simulink model "PWMinverter"  (Simulink 7.3)
settings: Solver=ode23tb  StartTime=0.0  StopTime=0.1  MaxStep=1e-5  RelTol=1e-3
libraries: powerlib x11, simulink x2
settings Model: Creator=viswam  LastModifiedBy=viswam
settings SolverCC: InitialStep=1e-6
settings OptimizationCC: InitFltsAndDblsToZero=on
settings DebuggingCC: SaveWithParameterizedLinksMsg=none  SignalResolutionControl=TryResolveAllWithWarning  MultiTaskDSMMsg=warning  MultiTaskCondExecSysMsg=none
settings RTWCC: IncludeERTFirstTime=on
settings GRTTargetCC: TargetFcnLib=ansi_tfl_tmw.mat

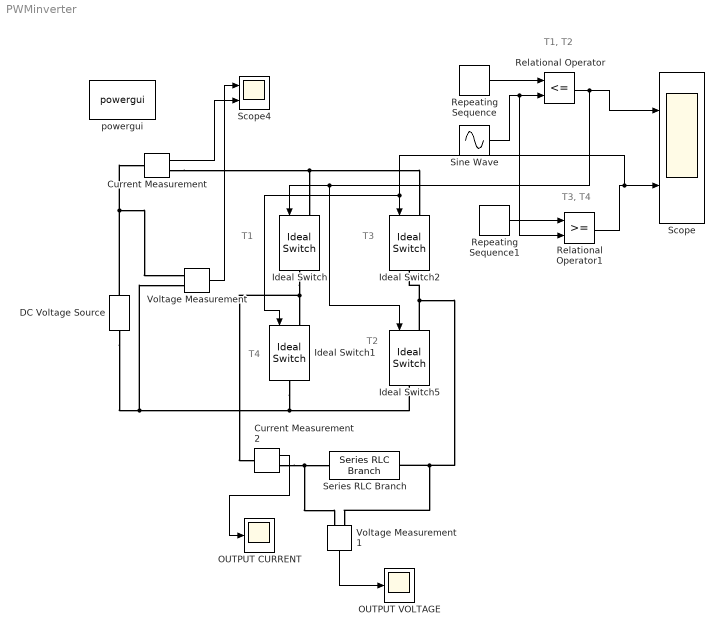
== system PWMinverter ==
  note: T1
  note: T2
  note: T3
  note: T4
  note: T1, T2
  note: T3, T4
  Current Measurement : powerlib/Measurements/Current Measurement  DialogController=POWERSYS.PowerSysDialog  SystemSampleTime=-1  PhasorSimulation=off  OutputType=Complex  PSBequivalent=0
  Current Measurement2 : powerlib/Measurements/Current Measurement  DialogController=POWERSYS.PowerSysDialog  SystemSampleTime=-1  PhasorSimulation=off  OutputType=Complex  PSBequivalent=0
  DC Voltage Source : powerlib/Electrical Sources/DC Voltage Source  DialogController=POWERSYS.PowerSysDialog  SystemSampleTime=-1  Amplitude=300  Measurements=None
  Ideal Switch{,1..2,5} (4 alike) : powerlib/Power Electronics/Ideal Switch  DialogController=POWERSYS.PowerSysDialog  SystemSampleTime=-1  Ron=0.001  Lon=0  IC=0  Rs=1e5  Cs=inf  Measurements=off
  OUTPUT CURRENT : Scope
      settings: TimeRange=0.04  YMin=-50  YMax=50  SaveName=outputcurrent
  OUTPUT VOLTAGE : Scope
      settings: TimeRange=0.04  YMin=-500  YMax=500  SaveName=outputvoltage
  Relational Operator : RelationalOperator  Operator=<=  LogicOutDataTypeMode=boolean  OutDataTypeStr=boolean
  Relational Operator1 : RelationalOperator  LogicOutDataTypeMode=boolean  OutDataTypeStr=boolean
  Repeating Sequence : simulink/Sources/Repeating Sequence  SystemSampleTime=-1  rep_seq_t=[0 0.5e-3 1e-3]  rep_seq_y=[0 1 0]
  Repeating Sequence1 : simulink/Sources/Repeating Sequence  SystemSampleTime=-1  rep_seq_t=[0 0.5e-3 1e-3]  rep_seq_y=[-1 0 -1]
  Scope : Scope  NumInputPorts=2
      settings: TimeRange=0.04  YMin=-5~-5  YMax=5~5
  Scope4 : Scope  NumInputPorts=2
      settings: TimeRange=0.04  YMin=-5~-5  YMax=5~5  SaveName=ScopeData4
  Series RLC Branch : powerlib/Elements/Series RLC Branch  DialogController=POWERSYS.PowerSysDialog  PhysicalDomain=powersysdomain  SubClassName=unknown  LeftPortType=p1  RightPortType=p1  LConnTagsString=__new0  RConnTagsString=__new0  BranchType=R  Resistance=10  Inductance=1e-3  SetiL0=off  InitialCurrent=0  Capacitance=1e-6  Setx0=off  InitialVoltage=0  Measurements=None
  Sine Wave : Sin  Amplitude=1  Bias=0  Frequency=2*pi*50  Phase=0  Samples=10  SampleTime=0  Offset=0
  Voltage Measurement : powerlib/Measurements/Voltage Measurement  DialogController=POWERSYS.PowerSysDialog  SystemSampleTime=-1  PhasorSimulation=off  OutputType=Complex  PSBequivalent=0
  Voltage Measurement1 : powerlib/Measurements/Voltage Measurement  DialogController=POWERSYS.PowerSysDialog  SystemSampleTime=-1  PhasorSimulation=off  OutputType=Complex  PSBequivalent=0
  powergui : powerlib/powergui  Priority=1  SystemSampleTime=-1  SimulationMode=Continuous  SampleTime=50e-6  frequency=60  SPID=off  DisableSnubberDevices=off  DisableRonSwitches=off  DisableVfSwitches=off  SwTol=0  Interpol=off  frequencyindice=0  echomessages=off  HookPort=off  DisplayEquations=off  FunctionMessages=off  EnableUseOfTLC=off  x0status=blocks  RestoreLinks=warning  Frange=[0:2:500]  Ylog=off  Xlog=on  ShowGrid=off  save=off  variable=ZData  ZoomFFT=on  StartTime=0.0  cycles=1  DisplayStyle=1  fundamental=60  FreqAxis=off  MaxFrequency=1000  frequencyindicesteady=1  RmsSteady=1  display=off  Ts=0  methode=off
  wires:
  Voltage Measurement/1 -> Scope4/1
  Current Measurement/1 -> Scope4/2
  Voltage Measurement1/1 -> OUTPUT VOLTAGE/1
  Current Measurement2/1 -> OUTPUT CURRENT/1
  Repeating Sequence/1 -> Relational Operator/1
  Sine Wave/1 -> Relational Operator/2, Relational Operator1/2
  Repeating Sequence1/1 -> Relational Operator1/1
  Relational Operator/1 -> Scope/1, Ideal Switch/1, Ideal Switch5/1
  Relational Operator1/1 -> Scope/2, Ideal Switch2/1, Ideal Switch1/1
  connections:
  Ideal Switch/RConn1 -- Ideal Switch1/LConn1 -- Current Measurement2/LConn1
  Ideal Switch5/LConn1 -- Ideal Switch2/RConn1 -- Series RLC Branch/LConn1 -- Voltage Measurement1/LConn2
  DC Voltage Source/LConn1 -- Voltage Measurement/LConn2 -- Ideal Switch5/RConn1 -- Ideal Switch1/RConn1
  Current Measurement2/RConn1 -- Series RLC Branch/RConn1 -- Voltage Measurement1/LConn1
  DC Voltage Source/RConn1 -- Current Measurement/LConn1 -- Voltage Measurement/LConn1
  Current Measurement/RConn1 -- Ideal Switch2/LConn1 -- Ideal Switch/LConn1
